simulink model "integrate"  (Simulink 8.3)
settings: Solver=ode3  StartTime=0.0  StopTime=simulation_time  FixedStep=dt  RelTol=1e-5
values from neighbouring files (symbols this model uses):
  k = 3    [test.m]    (also in test_2.m = 2)
  T = 5    [test.m]    (also in test_2.m = 10)
  w = omega(i)    [test.m]    (also in test_2.m = w_1(j))
settings Model: Creator=Павел  LastModifiedBy=Павел
settings DataIOCC: LimitDataPoints=off  SignalLoggingSaveFormat=Dataset
settings DebuggingCC: UnderspecifiedInitializationDetection=Simplified  StateNameClashWarn=none
settings GRTTargetCC: CombineOutputUpdateFcns=on  GRTInterface=off

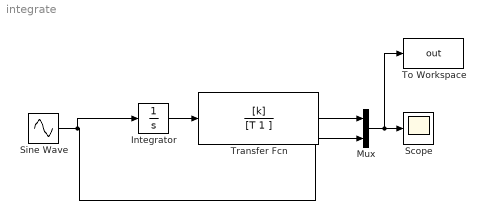
== system integrate ==
  Integrator : Integrator
  Mux : Mux  Inputs=2
  Scope : Scope
  Sine Wave : Sin  Frequency=w  SampleTime=0
  To Workspace : ToWorkspace  VariableName=out  SaveFormat=Structure With Time  SampleTime=-1
  Transfer Fcn : TransferFcn  Numerator=[k]  Denominator=[T 1 ]
  wires:
  Mux/1 -> To Workspace/1, Scope/1
  Sine Wave/1 -> Integrator/1, Mux/2
  Transfer Fcn/1 -> Mux/1
  Integrator/1 -> Transfer Fcn/1
